simulink model "GPSSmoothingEstimationVerification"  (R2018a)
settings: Solver=FixedStepAuto  StartTime=0.0  StopTime=120  FixedStep=0.001  RelTol=1e-3
undefined symbols (not defined in the file): magnitude, SkywalkerX8
libraries: sharedTrackingLibrary x1, dspmtrx3 x1
settings Model: Creator=David  LastModifiedBy=David

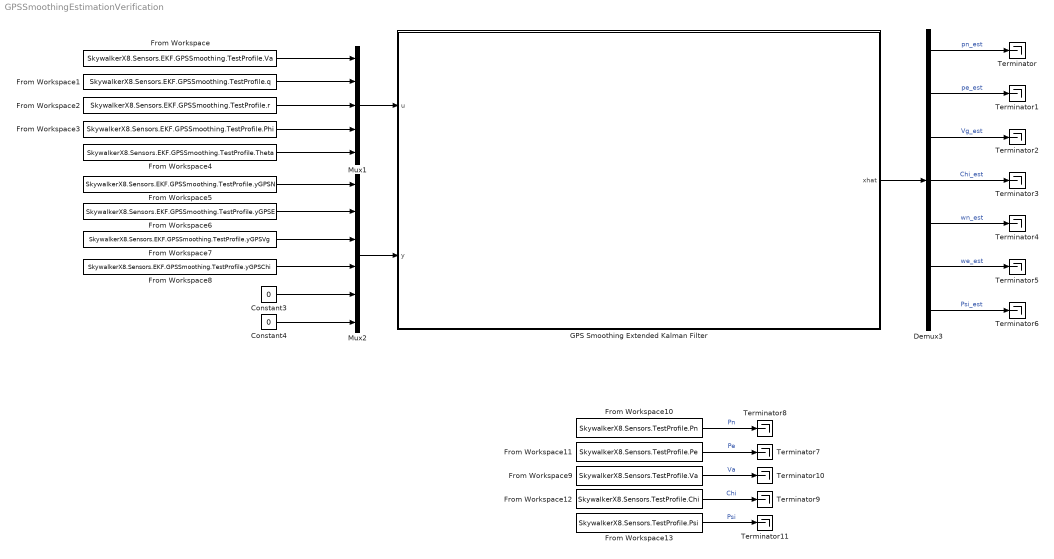
== system GPSSmoothingEstimationVerification ==
  Constant3 : Constant  Value=0
  Constant4 : Constant  Value=0
  Demux3 : Demux  Outputs=7
  From Workspace : FromWorkspace  VariableName=SkywalkerX8.Sensors.EKF.GPSSmoothing.TestProfile.Va  Interpolate=off  OutputAfterFinalValue=Holding final value
  From Workspace1 : FromWorkspace  VariableName=SkywalkerX8.Sensors.EKF.GPSSmoothing.TestProfile.q  Interpolate=off  OutputAfterFinalValue=Holding final value
  From Workspace10 : FromWorkspace  VariableName=SkywalkerX8.Sensors.TestProfile.Pn  Interpolate=off  OutputAfterFinalValue=Holding final value
  From Workspace11 : FromWorkspace  VariableName=SkywalkerX8.Sensors.TestProfile.Pe  Interpolate=off  OutputAfterFinalValue=Holding final value
  From Workspace12 : FromWorkspace  VariableName=SkywalkerX8.Sensors.TestProfile.Chi  Interpolate=off  OutputAfterFinalValue=Holding final value
  From Workspace13 : FromWorkspace  VariableName=SkywalkerX8.Sensors.TestProfile.Psi  Interpolate=off  OutputAfterFinalValue=Holding final value
  From Workspace2 : FromWorkspace  VariableName=SkywalkerX8.Sensors.EKF.GPSSmoothing.TestProfile.r  OutputAfterFinalValue=Holding final value
  From Workspace3 : FromWorkspace  VariableName=SkywalkerX8.Sensors.EKF.GPSSmoothing.TestProfile.Phi  Interpolate=off  OutputAfterFinalValue=Holding final value
  From Workspace4 : FromWorkspace  VariableName=SkywalkerX8.Sensors.EKF.GPSSmoothing.TestProfile.Theta  Interpolate=off  OutputAfterFinalValue=Holding final value
  From Workspace5 : FromWorkspace  VariableName=SkywalkerX8.Sensors.EKF.GPSSmoothing.TestProfile.yGPSN  Interpolate=off  OutputAfterFinalValue=Holding final value
  From Workspace6 : FromWorkspace  VariableName=SkywalkerX8.Sensors.EKF.GPSSmoothing.TestProfile.yGPSE  Interpolate=off  OutputAfterFinalValue=Holding final value
  From Workspace7 : FromWorkspace  VariableName=SkywalkerX8.Sensors.EKF.GPSSmoothing.TestProfile.yGPSVg  Interpolate=off  OutputAfterFinalValue=Holding final value
  From Workspace8 : FromWorkspace  VariableName=SkywalkerX8.Sensors.EKF.GPSSmoothing.TestProfile.yGPSChi  Interpolate=off  OutputAfterFinalValue=Holding final value
  From Workspace9 : FromWorkspace  VariableName=SkywalkerX8.Sensors.TestProfile.Va  Interpolate=off  OutputAfterFinalValue=Holding final value
  GPS Smoothing Extended Kalman Filter : Subsystem
      mask Display:
      | port_label('input', 1, '{\bf u} = [V_a, q, r, \Phi, \theta]', 'texMode', 'On')
      | port_label('input', 2, '{\bf y} = [y_{GPS_N}, y_{GPS_E}, y_{GPS_{V_g}}, y_{GPS_\chi}, y_{GPS_{wind_N}}, y_{GPS_{wind_E}}]', 'texMode', 'On')
      | 
      | port_label('output', 1, '{\bf x_{est}} = [p_n, p_e, V_g, \chi, w_n, w_e, \psi]', 'texMode', 'On')
  Mux1 : Mux  Inputs=5
  Mux2 : Mux  Inputs=6
  Terminator{,1..11} (12 alike) : Terminator
  wires:
  Demux3/2 -> Terminator1/1  "pe_est"
  Demux3/1 -> Terminator/1  "pn_est"
  Mux1/1 -> GPS Smoothing Extended Kalman Filter/1(u)
  Demux3/5 -> Terminator4/1  "wn_est"
  Demux3/3 -> Terminator2/1  "Vg_est"
  Demux3/6 -> Terminator5/1  "we_est"
  Mux2/1 -> GPS Smoothing Extended Kalman Filter/2(y)
  GPS Smoothing Extended Kalman Filter/1(xhat) -> Demux3/1
  Demux3/4 -> Terminator3/1  "Chi_est"
  Constant3/1 -> Mux2/5
  Demux3/7 -> Terminator6/1  "Psi_est"
  Constant4/1 -> Mux2/6
  From Workspace/1 -> Mux1/1
  From Workspace1/1 -> Mux1/2
  From Workspace2/1 -> Mux1/3
  From Workspace3/1 -> Mux1/4
  From Workspace4/1 -> Mux1/5
  From Workspace5/1 -> Mux2/1
  From Workspace6/1 -> Mux2/2
  From Workspace7/1 -> Mux2/3
  From Workspace8/1 -> Mux2/4
  From Workspace10/1 -> Terminator8/1  "Pn"
  From Workspace11/1 -> Terminator7/1  "Pe"
  From Workspace12/1 -> Terminator9/1  "Chi"
  From Workspace9/1 -> Terminator10/1  "Va"
  From Workspace13/1 -> Terminator11/1  "Psi"

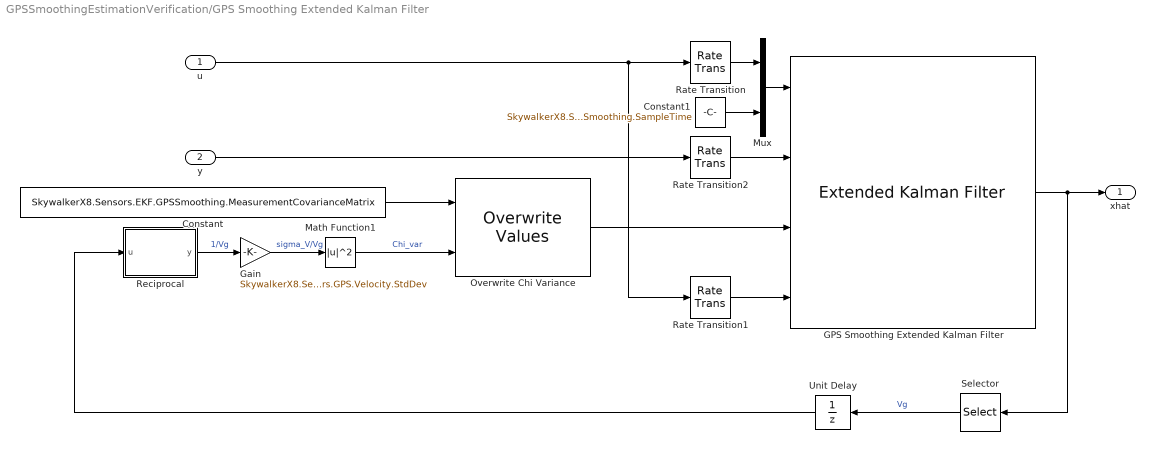
== system GPSSmoothingEstimationVerification/GPS Smoothing Extended Kalman Filter ==
  u : Inport  PortDimensions=5
  y : Inport  Port=2  PortDimensions=6
  Constant : Constant  Value=SkywalkerX8.Sensors.EKF.GPSSmoothing.MeasurementCovarianceMatrix
  Constant1 : Constant  Value=SkywalkerX8.Sensors.EKF.GPSSmoothing.SampleTime
  GPS Smoothing Extended Kalman Filter : sharedTrackingLibrary/Extended Kalman Filter  StateTransitionFcn=GPSSmoothingTransitionEstimate  HasStateTransitionJacobianFcn=on  StateTransitionJacobianFcn=GPSSmoothingTransitionEstimate_Jacobian  HasAdditiveProcessNoise=Additive  ProcessNoise=SkywalkerX8.Sensors.EKF.GPSSmoothing.ProcessCovarianceMatrix  HasTimeVaryingProcessNoise=off  HasStateTransitionFcnExtraArgument=1  InitialState=SkywalkerX8.Sensors.EKF.GPSSmoothing.InitialState  InitialStateCovariance=SkywalkerX8.Sensors.EKF.GPSSmoothing.InitialStateCovarianceMatrix  MeasurementFcn1=GPSSmoothingMeasurementEstimate  HasMeasurementJacobianFcn1=on  MeasurementJacobianFcn1=GPSSmoothingMeasurementEstimate_Jacobian  HasMeasurementEnablePort1=off  HasAdditiveMeasurementNoise1=Additive  MeasurementNoise1=SkywalkerX8.Sensors.EKF.GPSSmoothing.MeasurementCovarianceMatrix  HasTimeVaryingMeasurementNoise1=on  HasMeasurementFcnExtraArgument1=1  MeasurementFcn2=myMeasurementFcn  HasMeasurementJacobianFcn2=off  HasMeasurementEnablePort2=off  HasAdditiveMeasurementNoise2=Additive  MeasurementNoise2=1  HasTimeVaryingMeasurementNoise2=off  HasMeasurementFcnExtraArgument2=0  MeasurementFcn3=myMeasurementFcn  HasMeasurementJacobianFcn3=off  HasMeasurementEnablePort3=off  HasAdditiveMeasurementNoise3=Additive  MeasurementNoise3=1  HasTimeVaryingMeasurementNoise3=off  HasMeasurementFcnExtraArgument3=0  MeasurementFcn4=myMeasurementFcn  HasMeasurementJacobianFcn4=off  HasMeasurementEnablePort4=off  HasAdditiveMeasurementNoise4=Additive  MeasurementNoise4=1  HasTimeVaryingMeasurementNoise4=off  HasMeasurementFcnExtraArgument4=0  MeasurementFcn5=myMeasurementFcn  HasMeasurementJacobianFcn5=off  HasMeasurementEnablePort5=off  HasAdditiveMeasurementNoise5=Additive  MeasurementNoise5=1  HasTimeVaryingMeasurementNoise5=off  HasMeasurementFcnExtraArgument5=0  EnableMultirate=on  StateTransitionFcnSampleTime=SkywalkerX8.Sensors.EKF.GPSSmoothing.StateTransitionSampleTime  MeasurementFcn1SampleTime=SkywalkerX8.Sensors.EKF.GPSSmoothing.MeasurementSampleTime  MeasurementFcn2SampleTime=1  MeasurementFcn3SampleTime=1  MeasurementFcn4SampleTime=1  MeasurementFcn5SampleTime=1  UseCurrentEstimator=on  OutputStateCovariance=off  DataType=double  SampleTime=SkywalkerX8.Sensors.EKF.GPSSmoothing.SampleTime  NumberOfMeasurements=1
      settings: SourceProductName=Control System Toolbox  SourceProductBaseCode=CT
  Gain : Gain  Gain=SkywalkerX8.Sensors.GPS.Velocity.StdDev
  Math Function1 : Math  Operator=magnitude^2  SaturateOnIntegerOverflow=on
  Mux : Mux  Inputs=2
  Overwrite Chi Variance : dspmtrx3/Overwrite Values  OverWriteDiag=Submatrix  valFrom2ndIP=Second input port  ConstValue=0  RowSpan=One row  RowStartMode=Index  RowStartIndex=4  RowEndMode=Last  RowEndIndex=1  ColSpan=One column  ColStartMode=First  ColStartIndex=1  ColEndMode=Last  ColEndIndex=1  DiagSpan=Range of elements  DiagStartMode=Index  DiagStartIndex=2  DiagEndMode=Index  DiagEndIndex=4
      settings: SourceProductName=DSP System Toolbox  SourceProductBaseCode=DS
  Rate Transition : RateTransition  InitialCondition=SkywalkerX8.Sensors.EKF.GPSSmoothing.InitialInput  OutPortSampleTime=SkywalkerX8.Sensors.EKF.GPSSmoothing.StateTransitionSampleTime
  Rate Transition1 : RateTransition  InitialCondition=SkywalkerX8.Sensors.EKF.GPSSmoothing.InitialInput  OutPortSampleTime=SkywalkerX8.Sensors.EKF.GPSSmoothing.MeasurementSampleTime
  Rate Transition2 : RateTransition  InitialCondition=SkywalkerX8.Sensors.EKF.GPSSmoothing.InitialMeasurement  OutPortSampleTime=SkywalkerX8.Sensors.EKF.GPSSmoothing.MeasurementSampleTime
  Reciprocal : MATLAB Function  TreatAsAtomicUnit=on
  Selector : Selector  InputPortWidth=7  IndexOptions=Index vector (dialog)  Indices=3  OutputSizes=1
  Unit Delay : UnitDelay  InitialCondition=SkywalkerX8.Sensors.EKF.GPSSmoothing.InitialState(3)  SampleTime=SkywalkerX8.Sensors.EKF.GPSSmoothing.MeasurementSampleTime
  xhat : Outport
  wires:
  y/1 -> Rate Transition2/1
  GPS Smoothing Extended Kalman Filter/1 -> Selector/1, xhat/1
  Reciprocal/1(y) -> Gain/1  "1/Vg"
  Gain/1 -> Math Function1/1  "sigma_V/Vg"
  Math Function1/1 -> Overwrite Chi Variance/2  "Chi_var"
  Constant/1 -> Overwrite Chi Variance/1
  Overwrite Chi Variance/1 -> GPS Smoothing Extended Kalman Filter/3
  u/1 -> Rate Transition1/1, Rate Transition/1
  Selector/1 -> Unit Delay/1  "Vg"
  Unit Delay/1 -> Reciprocal/1(u)
  Rate Transition1/1 -> GPS Smoothing Extended Kalman Filter/4
  Rate Transition2/1 -> GPS Smoothing Extended Kalman Filter/2
  Rate Transition/1 -> Mux/1
  Mux/1 -> GPS Smoothing Extended Kalman Filter/1
  Constant1/1 -> Mux/2

== matlab function GPSSmoothingEstimationVerification/GPS Smoothing Extended Kalman Filter/Reciprocal ==
  data: u input; y output
function y = reciprocal(u)

    if (u ~= 0)
       y = 1/u;
    else
       y = 1E06; 
    end

end
